simulink model "BremsenOhneMitABS_Pacejka"  (Simulink 9.2)
settings: Solver=ode45  StartTime=0.0  StopTime=4  FixedStep=0.01  RelTol=1e-9  AbsTol=1e-9  EnableMultiTasking=on
values from neighbouring files (symbols this model uses):
  A = 2    [Bremsen_abs.m]
  cw = 0.3    [Bremsen_abs.m]
  g = 9.81    [Bremsen_abs.m]
  JR = 0.8    [Bremsen_abs.m]
  m = 1500    [Bremsen_abs.m]
  mfB = 5    [Bremsen_abs.m]
  mfC = 2.3    [Bremsen_abs.m]
  mfD = 1.05    [Bremsen_abs.m]
  mfE = 1.04    [Bremsen_abs.m]
  rho = 1.2    [Bremsen_abs.m]
  rR = 0.3    [Bremsen_abs.m]
  v0 = 100/3.6    (= 27.7777777778)    [Bremsen_abs.m]
settings Model: Creator=wang  LastModifiedBy=wang  ExtModeTrigMode=oneshot  ExtModeArmWhenConnect=off
settings SolverCC: AutoScaleAbsTol=off
settings DataIOCC: LimitDataPoints=off
settings OptimizationCC: BooleanDataType=off  ExpressionDepthLimit=2147483647  InitFltsAndDblsToZero=on
settings DebuggingCC: SaveWithParameterizedLinksMsg=none  SignalResolutionControl=TryResolveAllWithWarning  MultiTaskDSMMsg=warning  MultiTaskCondExecSysMsg=none
settings HardwareCC: TargetUnknown=on
settings SFSimCC: SimUseLocalCustomCode=on
settings RTWCC: RTWUseLocalCustomCode=on
settings GRTTargetCC: ModelReferenceCompliant=off  ParMdlRefBuildCompliant=off  CompOptLevelCompliant=off  ConcurrentExecutionCompliant=off  GeneratePreprocessorConditionals=Use local settings  MatFileLogging=off  MATLABClassNameForMDSCustomization=Simulink.SoftwareTarget.TargetSpecificTriggerConfigurationBase
settings ConfigComp: CovExternalEMLEnable=on

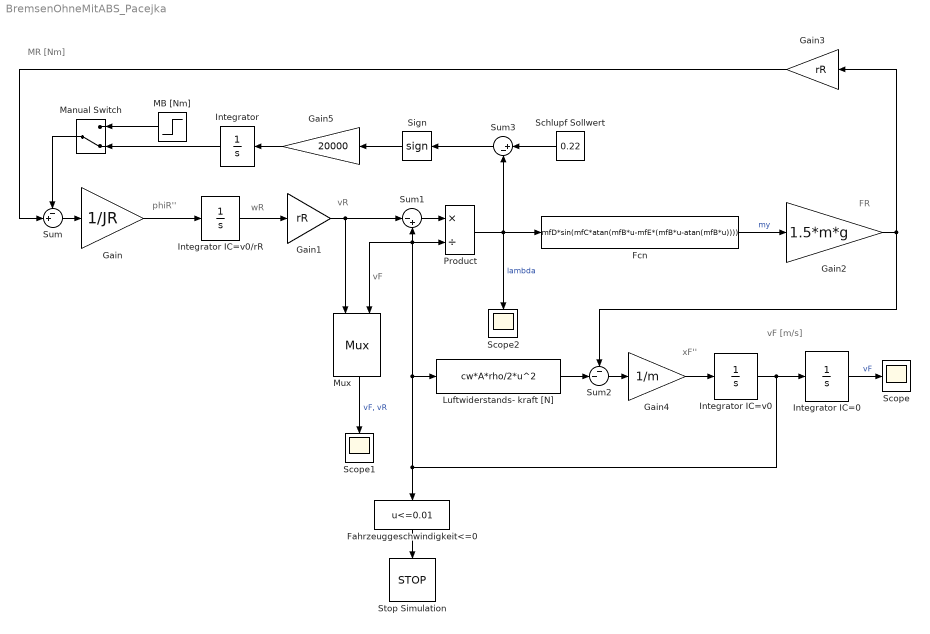
== system BremsenOhneMitABS_Pacejka ==
  note: phiR''
  note: wR
  note: FR
  note: MR [Nm]
  note: xF''
  note: vF
      | [m/s]
  note: vR
  note: vF
  Fahrzeuggeschwindigkeit<=0 : Fcn  Expr=u<=0.01
  Fcn : Fcn  Expr=mfD*sin(mfC*atan(mfB*u-mfE*(mfB*u-atan(mfB*u))))
  Gain : Gain  Gain=1/JR  SaturateOnIntegerOverflow=on  OutDataTypeStr=Inherit: Same as input  ParamDataTypeStr=Inherit: Same as input
  Gain1 : Gain  Gain=rR  SaturateOnIntegerOverflow=on  OutDataTypeStr=Inherit: Same as input  ParamDataTypeStr=Inherit: Same as input
  Gain2 : Gain  Gain=1.5*m*g  SaturateOnIntegerOverflow=on  OutDataTypeStr=Inherit: Same as input  ParamDataTypeStr=Inherit: Same as input
  Gain3 : Gain  Gain=rR  SaturateOnIntegerOverflow=on  OutDataTypeStr=Inherit: Same as input  ParamDataTypeStr=Inherit: Same as input
  Gain4 : Gain  Gain=1/m  SaturateOnIntegerOverflow=on  OutDataTypeStr=Inherit: Same as input  ParamDataTypeStr=Inherit: Same as input
  Gain5 : Gain  Gain=20000  SaturateOnIntegerOverflow=on  OutDataTypeStr=Inherit: Same as input  ParamDataTypeStr=Inherit: Same as input
  Integrator : Integrator  LimitOutput=on  LowerSaturationLimit=0
  Integrator IC=0 : Integrator  LimitOutput=on  LowerSaturationLimit=0
  Integrator IC=v0 : Integrator  InitialCondition=v0  LimitOutput=on  LowerSaturationLimit=0
  Integrator IC=v0/rR : Integrator  InitialCondition=v0/rR  LimitOutput=on  LowerSaturationLimit=0
  Luftwiderstands- kraft [N] : Fcn  Expr=cw*A*rho/2*u^2
  MB [Nm] : Step  Time=0  After=5355  SampleTime=0
  Manual Switch : ManualSwitch  CurrentSetting=0
  Mux : Mux  Inputs=2
      settings: DisplayOption=signals
  Product : Product  Inputs=*/  SaturateOnIntegerOverflow=on  RndMeth=Zero  InputSameDT=on  OutDataTypeStr=Inherit: Same as first input
  Schlupf Sollwert : Constant  Value=0.22
  Scope : Scope
  Scope1 : Scope
  Scope2 : Scope
  Sign : Signum
  Stop Simulation : Stop
  Sum : Sum  Inputs=-+|  SaturateOnIntegerOverflow=on  InputSameDT=on  OutDataTypeStr=Inherit: Same as first input
  Sum1 : Sum  Inputs=|-+  SaturateOnIntegerOverflow=on  InputSameDT=on  OutDataTypeStr=Inherit: Same as first input
  Sum2 : Sum  Inputs=--|  SaturateOnIntegerOverflow=on  InputSameDT=on  OutDataTypeStr=Inherit: Same as first input
  Sum3 : Sum  Inputs=|+-  SaturateOnIntegerOverflow=on  InputSameDT=on  OutDataTypeStr=Inherit: Same as first input
  wires:
  MB [Nm]/1 -> Manual Switch/1
  Sum/1 -> Gain/1
  Gain/1 -> Integrator IC=v0/rR/1
  Integrator IC=v0/rR/1 -> Gain1/1
  Sum1/1 -> Product/1
  Fcn/1 -> Gain2/1  "my"
  Gain3/1 -> Sum/2
  Luftwiderstands- kraft [N]/1 -> Sum2/2
  Sum2/1 -> Gain4/1
  Gain4/1 -> Integrator IC=v0/1
  Integrator IC=v0/1 -> Integrator IC=0/1, Luftwiderstands- kraft [N]/1, Sum1/2, Mux/2, Product/2, Fahrzeuggeschwindigkeit<=0/1
  Integrator IC=0/1 -> Scope/1  "vF"
  Product/1 -> Fcn/1, Scope2/1, Sum3/2  "lambda"
  Fahrzeuggeschwindigkeit<=0/1 -> Stop Simulation/1
  Gain1/1 -> Sum1/1, Mux/1
  Mux/1 -> Scope1/1  "vF, vR"
  Gain2/1 -> Gain3/1, Sum2/1
  Manual Switch/1 -> Sum/1
  Schlupf Sollwert/1 -> Sum3/1
  Gain5/1 -> Integrator/1
  Sign/1 -> Gain5/1
  Integrator/1 -> Manual Switch/2
  Sum3/1 -> Sign/1
